simulink model "LPV_control"  (R2023a)
settings: Solver=VariableStepAuto  StartTime=0.0  StopTime=30  RelTol=1e-3
values from neighbouring files (symbols this model uses):
  Ad = [-1/t_beta 0 ... (first row only)    [calc_KMax.m]    (also in calc_Kmin.m; modelo.m)
  C = [1 0 ... (first row only)    [modelo.m]
  D = [0 0;0 0]    [modelo.m]
  Ed = [k_beta/t_beta ... (first row only)    [calc_KMax.m]    (also in calc_Kmin.m; modelo.m)
  x0 = [0, 0]    [modelo.m]
undefined symbols (not defined in the file or in its folder): calc_A, calc_B, calc_E, calc_inv_B, sigbuilder_block
settings Model: Creator=Ferna  LastModifiedBy=Ferna

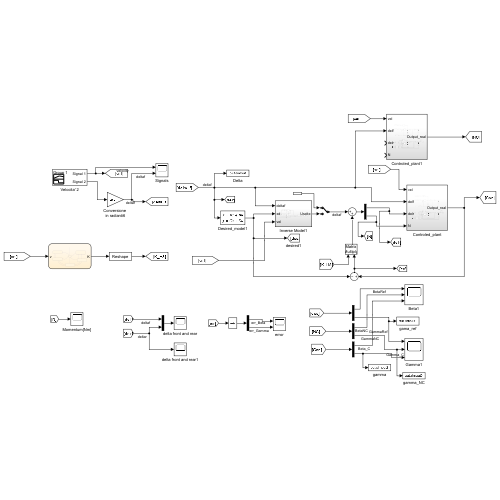
[thumbnail: Simulink's stored preview of the top-level diagram]
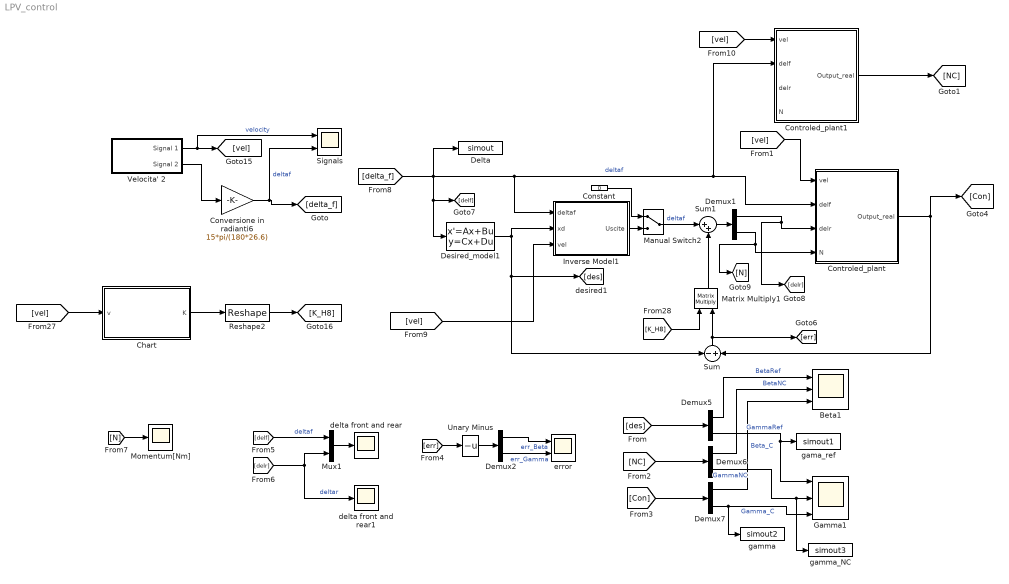
== system LPV_control ==
  Beta1 : Scope  NumInputPorts=3
  Chart : Stateflow chart  TreatAsAtomicUnit=on
  Constant : Constant  Value=0
  Controled_plant : Subsystem
  Controled_plant1 : Subsystem
  Conversione in radianti6 : Gain  Gain=15*pi/(180*26.6)
  Delta : ToWorkspace  VariableName=simout  SaveFormat=Timeseries  SampleTime=-1
  Demux{1..2,5..7} (5 alike) : Demux  Outputs=2
  Desired_model1 : StateSpace  A=Ad  B=Ed  C=[1,0;0,1]  D=zeros(2,1)  InitialCondition=0
  Gamma1 : Scope  NumInputPorts=3
  Inverse Model1 : Subsystem
  Manual Switch2 : ManualSwitch
  Matrix Multiply1 : Product  Multiplication=Matrix(*)
  Momentum[Nm] : Scope
  Mux1 : Mux  Inputs=2
  Reshape2 : Reshape  OutputDimensionality=Customize  OutputDimensions=[2,2]
  Signals : Scope  NumInputPorts=2
  Sum : Sum  Inputs=-|+
  Sum1 : Sum  Inputs=|++
  Unary Minus : UnaryMinus
  Velocita' 2 : Subsystem  Tag=STV Subsys  LoadFcn=sigbuilder_block('load');  StartFcn=sigbuilder_block('start');  StopFcn=sigbuilder_block('stop');  ClipboardFcn=sigbuilder_block('clipboard');  mask(Sigbuilder block){tuvar=[0:10]}
      mask help: Simulink:masks:SigbuilderBlock_MD
      mask init:
      | if ~strcmp(get_param(bdroot(gcbh),'SimulationStatus'),'stopped') tuvar = sigbuilder_block('maskInit'); end
      settings: CopyFcn=sigbuilder_block('copy');  DeleteFcn=sigbuilder_block('delete');  ModelCloseFcn=sigbuilder_block('modelClose');  PreSaveFcn=sigbuilder_block('preSave');  PauseFcn=sigbuilder_block('pause');  ContinueFcn=sigbuilder_block('continue');  NameChangeFcn=sigbuilder_block('namechange');  OpenFcn=sigbuilder_block('open',[5.4 36 1141.2 516.6 ]);  CloseFcn=sigbuilder_block('close');
      mask Display: plot(0, 0, 100, 100,[2, 2, 32, 32, 2], [68, 8, 8, 68, 68],[32, 2], [38, 38], [32, 19, 2],[53, 60, 44], [32, 17, 17, 2],[16, 16, 31, 31]);txt = getActiveGroup(gcbh);text(2, 100, txt,'verticalAlignment', 'top');
  delta front and rear : Scope
  delta front and rear1 : Scope
  error : Scope  NumInputPorts=2
  gama_ref : ToWorkspace  VariableName=simout1  SaveFormat=Timeseries  SampleTime=-1
  gamma : ToWorkspace  VariableName=simout2  SaveFormat=Timeseries  SampleTime=-1
  gamma_NC : ToWorkspace  VariableName=simout3  SaveFormat=Timeseries  SampleTime=-1
  wires:
  Conversione in radianti6/1 -> Signals/2, [delta_f]  "deltaf"
  Velocita' 2/2(Signal 2) -> Conversione in radianti6/1
  Demux5/2 -> gama_ref/1, Gamma1/1  "GammaRef"
  [N] -> Momentum[Nm]/1
  [delf] -> Mux1/1  "deltaf"
  Demux2/2 -> error/2  "err_Gamma"
  [delta_f] -> [delf], Desired_model1/1, Delta/1, Inverse Model1/1(deltaf), Controled_plant1/2(delf), Controled_plant/2(delf)  "deltaf"
  Demux2/1 -> error/1  "err_Beta"
  Mux1/1 -> delta front and rear/1
  Unary Minus/1 -> Demux2/1
  Sum1/1 -> Demux1/1
  Demux5/1 -> Beta1/1  "BetaRef"
  Demux6/1 -> Beta1/2  "BetaNC"
  [Con] -> Demux7/1
  [err] -> Unary Minus/1
  Demux1/1 -> [delr], Controled_plant/3(delr)
  [NC] -> Demux6/1
  Desired_model1/1 -> Inverse Model1/2(xd), Sum/1, [des]
  Demux1/2 -> [N], Controled_plant/4(N)
  Demux7/2 -> gamma/1, Gamma1/3  "Gamma_C"
  [delr] -> Mux1/2, delta front and rear1/1  "deltar"
  Demux7/1 -> Beta1/3  "Beta_C"
  [des] -> Demux5/1
  Controled_plant/1(Output_real) -> [Con], Sum/2
  Demux6/2 -> gamma_NC/1, Gamma1/2  "GammaNC"
  [vel] -> Controled_plant/1(vel)
  Velocita' 2/1(Signal 1) -> Signals/1, [vel]  "velocity"
  [vel] -> Inverse Model1/3(vel)
  Inverse Model1/1(Uscite) -> Manual Switch2/2
  Constant/1 -> Manual Switch2/1
  Manual Switch2/1 -> Sum1/1  "deltaf"
  Reshape2/1 -> [K_H8]
  [vel] -> Chart/1(v)
  Chart/1(K) -> Reshape2/1
  [K_H8] -> Matrix Multiply1/1
  Sum/1 -> Matrix Multiply1/2, [err]
  Matrix Multiply1/1 -> Sum1/2
  Controled_plant1/1(Output_real) -> [NC]
  [vel] -> Controled_plant1/1(vel)

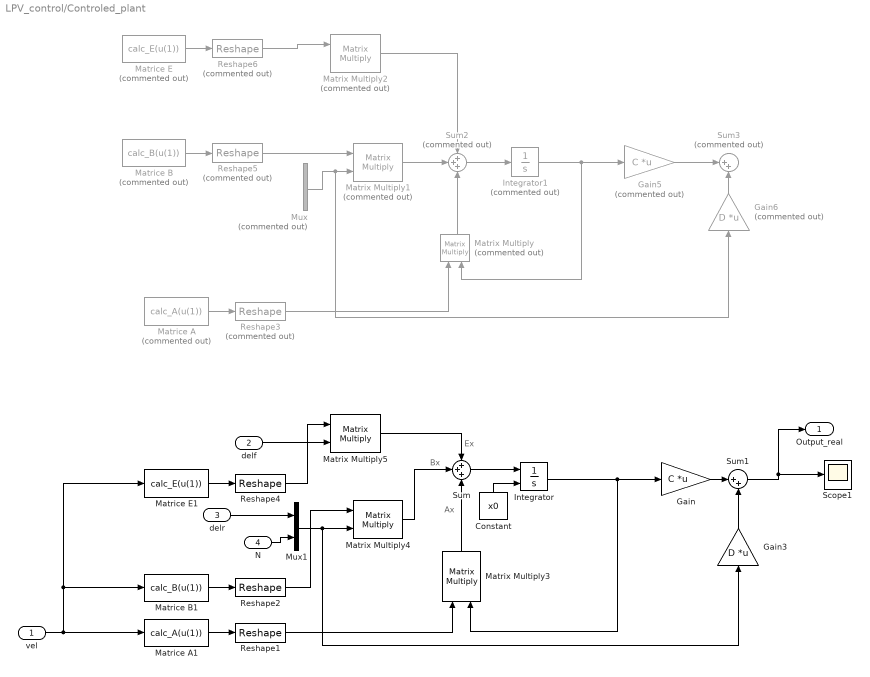
== system LPV_control/Controled_plant ==
  note: Ex
  note: Bx
  note: Ax
  vel : Inport
  delf : Inport  Port=2
  delr : Inport  Port=3
  N : Inport  Port=4
  Constant : Constant  Value=x0
  Gain : Gain  Gain=C  Multiplication=Matrix(K*u)
  Gain3 : Gain  Gain=D  Multiplication=Matrix(K*u)
  Gain5 : Gain  Commented=on  Gain=C  Multiplication=Matrix(K*u)
  Gain6 : Gain  Commented=on  Gain=D  Multiplication=Matrix(K*u)
  Integrator : Integrator  InitialConditionSource=external
  Integrator1 : Integrator  Commented=on  InitialCondition=x0
  Matrice A : MATLABFcn  Commented=on  MATLABFcn=calc_A(u(1))
  Matrice A1 : MATLABFcn  MATLABFcn=calc_A(u(1))
  Matrice B : MATLABFcn  Commented=on  MATLABFcn=calc_B(u(1))
  Matrice B1 : MATLABFcn  MATLABFcn=calc_B(u(1))
  Matrice E : MATLABFcn  Commented=on  MATLABFcn=calc_E(u(1))
  Matrice E1 : MATLABFcn  MATLABFcn=calc_E(u(1))
  Matrix Multiply : Product  Commented=on  Multiplication=Matrix(*)
  Matrix Multiply1 : Product  Commented=on  Multiplication=Matrix(*)
  Matrix Multiply2 : Product  Commented=on  Multiplication=Matrix(*)
  Matrix Multiply3 : Product  Multiplication=Matrix(*)
  Matrix Multiply4 : Product  Multiplication=Matrix(*)
  Matrix Multiply5 : Product  Multiplication=Matrix(*)
  Mux : Mux  Commented=on  Inputs=2
  Mux1 : Mux  Inputs=2
  Reshape1 : Reshape  OutputDimensionality=Customize  OutputDimensions=[2,2]
  Reshape2 : Reshape  OutputDimensionality=Customize  OutputDimensions=[2,2]
  Reshape3 : Reshape  Commented=on  OutputDimensionality=Customize  OutputDimensions=[2,2]
  Reshape4 : Reshape  OutputDimensionality=Customize  OutputDimensions=[2,1]
  Reshape5 : Reshape  Commented=on  OutputDimensionality=Customize  OutputDimensions=[2,2]
  Reshape6 : Reshape  Commented=on  OutputDimensionality=Customize  OutputDimensions=[2,1]
  Scope1 : Scope
  Sum : Sum  Inputs=+++
  Sum1 : Sum  Inputs=|++
  Sum2 : Sum  Commented=on  Inputs=+++
  Sum3 : Sum  Commented=on  Inputs=|++
  Output_real : Outport
  wires:
  Matrice E/1 -> Reshape6/1
  Reshape6/1 -> Matrix Multiply2/1
  Matrix Multiply1/1 -> Sum2/2
  Mux/1 -> Gain6/1, Matrix Multiply1/2
  Reshape3/1 -> Matrix Multiply/1
  Matrice A/1 -> Reshape3/1
  Gain5/1 -> Sum3/1
  Gain6/1 -> Sum3/2
  Integrator1/1 -> Gain5/1, Matrix Multiply/2
  Sum2/1 -> Integrator1/1
  Matrix Multiply2/1 -> Sum2/1
  Matrix Multiply/1 -> Sum2/3
  Matrice B/1 -> Reshape5/1
  Reshape5/1 -> Matrix Multiply1/1
  Matrix Multiply3/1 -> Sum/3
  delf/1 -> Matrix Multiply5/2
  Mux1/1 -> Gain3/1, Matrix Multiply4/2
  Gain3/1 -> Sum1/2
  Reshape2/1 -> Matrix Multiply4/1
  Matrix Multiply5/1 -> Sum/1
  Matrice A1/1 -> Reshape1/1
  Matrice E1/1 -> Reshape4/1
  Gain/1 -> Sum1/1
  vel/1 -> Matrice A1/1, Matrice E1/1, Matrice B1/1
  Sum/1 -> Integrator/1
  Reshape4/1 -> Matrix Multiply5/1
  Matrix Multiply4/1 -> Sum/2
  Integrator/1 -> Matrix Multiply3/2, Gain/1
  delr/1 -> Mux1/1
  Reshape1/1 -> Matrix Multiply3/1
  Matrice B1/1 -> Reshape2/1
  Constant/1 -> Integrator/2
  Sum1/1 -> Output_real/1, Scope1/1
  N/1 -> Mux1/2

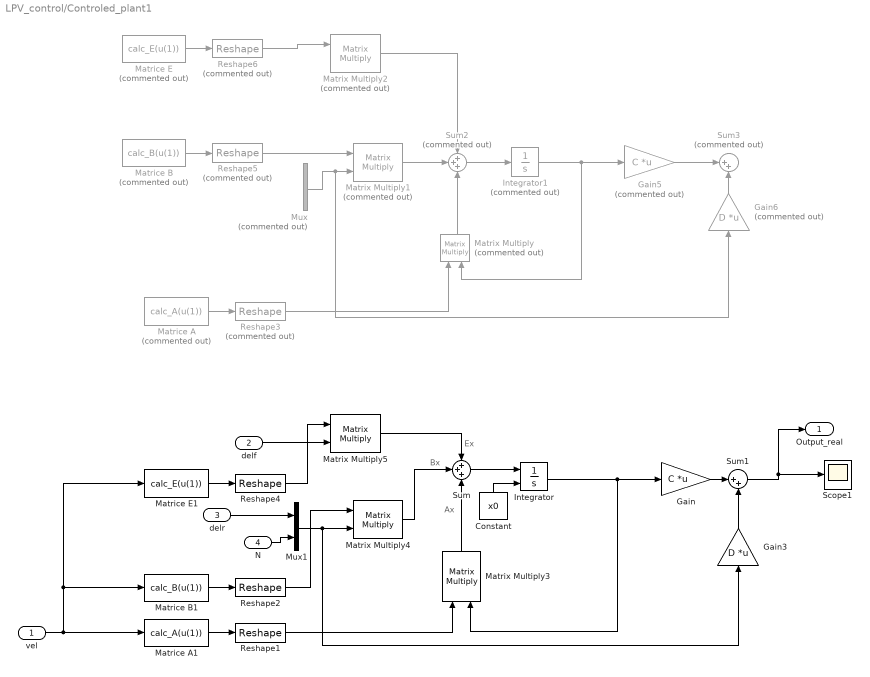
== system LPV_control/Controled_plant1 ==
  note: Ax
  note: Bx
  note: Ex
  vel : Inport
  delf : Inport  Port=2
  delr : Inport  Port=3
  N : Inport  Port=4
  Constant : Constant  Value=x0
  Gain : Gain  Gain=C  Multiplication=Matrix(K*u)
  Gain3 : Gain  Gain=D  Multiplication=Matrix(K*u)
  Gain5 : Gain  Commented=on  Gain=C  Multiplication=Matrix(K*u)
  Gain6 : Gain  Commented=on  Gain=D  Multiplication=Matrix(K*u)
  Integrator : Integrator  InitialConditionSource=external
  Integrator1 : Integrator  Commented=on  InitialCondition=x0
  Matrice A : MATLABFcn  Commented=on  MATLABFcn=calc_A(u(1))
  Matrice A1 : MATLABFcn  MATLABFcn=calc_A(u(1))
  Matrice B : MATLABFcn  Commented=on  MATLABFcn=calc_B(u(1))
  Matrice B1 : MATLABFcn  MATLABFcn=calc_B(u(1))
  Matrice E : MATLABFcn  Commented=on  MATLABFcn=calc_E(u(1))
  Matrice E1 : MATLABFcn  MATLABFcn=calc_E(u(1))
  Matrix Multiply : Product  Commented=on  Multiplication=Matrix(*)
  Matrix Multiply1 : Product  Commented=on  Multiplication=Matrix(*)
  Matrix Multiply2 : Product  Commented=on  Multiplication=Matrix(*)
  Matrix Multiply3 : Product  Multiplication=Matrix(*)
  Matrix Multiply4 : Product  Multiplication=Matrix(*)
  Matrix Multiply5 : Product  Multiplication=Matrix(*)
  Mux : Mux  Commented=on  Inputs=2
  Mux1 : Mux  Inputs=2
  Reshape1 : Reshape  OutputDimensionality=Customize  OutputDimensions=[2,2]
  Reshape2 : Reshape  OutputDimensionality=Customize  OutputDimensions=[2,2]
  Reshape3 : Reshape  Commented=on  OutputDimensionality=Customize  OutputDimensions=[2,2]
  Reshape4 : Reshape  OutputDimensionality=Customize  OutputDimensions=[2,1]
  Reshape5 : Reshape  Commented=on  OutputDimensionality=Customize  OutputDimensions=[2,2]
  Reshape6 : Reshape  Commented=on  OutputDimensionality=Customize  OutputDimensions=[2,1]
  Scope1 : Scope
  Sum : Sum  Inputs=+++
  Sum1 : Sum  Inputs=|++
  Sum2 : Sum  Commented=on  Inputs=+++
  Sum3 : Sum  Commented=on  Inputs=|++
  Output_real : Outport
  wires:
  N/1 -> Mux1/2
  Sum1/1 -> Scope1/1, Output_real/1
  Constant/1 -> Integrator/2
  Matrice B1/1 -> Reshape2/1
  Reshape1/1 -> Matrix Multiply3/1
  delr/1 -> Mux1/1
  Integrator/1 -> Gain/1, Matrix Multiply3/2
  Matrix Multiply4/1 -> Sum/2
  Reshape4/1 -> Matrix Multiply5/1
  Sum/1 -> Integrator/1
  vel/1 -> Matrice B1/1, Matrice E1/1, Matrice A1/1
  Gain/1 -> Sum1/1
  Matrice E1/1 -> Reshape4/1
  Matrice A1/1 -> Reshape1/1
  Matrix Multiply5/1 -> Sum/1
  Reshape2/1 -> Matrix Multiply4/1
  Gain3/1 -> Sum1/2
  Mux1/1 -> Matrix Multiply4/2, Gain3/1
  delf/1 -> Matrix Multiply5/2
  Matrix Multiply3/1 -> Sum/3
  Reshape5/1 -> Matrix Multiply1/1
  Matrice B/1 -> Reshape5/1
  Matrix Multiply/1 -> Sum2/3
  Matrix Multiply2/1 -> Sum2/1
  Sum2/1 -> Integrator1/1
  Integrator1/1 -> Matrix Multiply/2, Gain5/1
  Gain6/1 -> Sum3/2
  Gain5/1 -> Sum3/1
  Matrice A/1 -> Reshape3/1
  Reshape3/1 -> Matrix Multiply/1
  Mux/1 -> Matrix Multiply1/2, Gain6/1
  Matrix Multiply1/1 -> Sum2/2
  Reshape6/1 -> Matrix Multiply2/1
  Matrice E/1 -> Reshape6/1

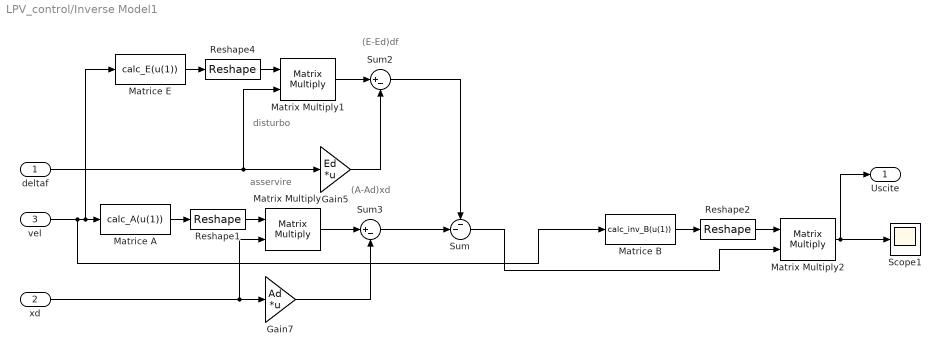
== system LPV_control/Inverse Model1 ==
  note: disturbo
  note: asservire
  note: (E-Ed)df
  note: (A-Ad)xd
  deltaf : Inport
  xd : Inport  Port=2  PortDimensions=2
  vel : Inport  Port=3  PortDimensions=1
  Gain5 : Gain  Gain=Ed  Multiplication=Matrix(K*u)
  Gain7 : Gain  Gain=Ad  Multiplication=Matrix(K*u)
  Matrice A : MATLABFcn  MATLABFcn=calc_A(u(1))
  Matrice B : MATLABFcn  MATLABFcn=calc_inv_B(u(1))
  Matrice E : MATLABFcn  MATLABFcn=calc_E(u(1))
  Matrix Multiply : Product  Multiplication=Matrix(*)
  Matrix Multiply1 : Product  Multiplication=Matrix(*)
  Matrix Multiply2 : Product  Multiplication=Matrix(*)
  Reshape1 : Reshape  OutputDimensionality=Customize  OutputDimensions=[2,2]
  Reshape2 : Reshape  OutputDimensionality=Customize  OutputDimensions=[2,2]
  Reshape4 : Reshape  OutputDimensionality=Customize  OutputDimensions=[2,1]
  Scope1 : Scope
  Sum : Sum  Inputs=--|
  Sum2 : Sum  Inputs=|+-
  Sum3 : Sum  Inputs=|+-
  Uscite : Outport
  wires:
  xd/1 -> Gain7/1, Matrix Multiply/2
  deltaf/1 -> Matrix Multiply1/2, Gain5/1
  Matrix Multiply1/1 -> Sum2/1
  Gain5/1 -> Sum2/2
  Gain7/1 -> Sum3/2
  Matrix Multiply/1 -> Sum3/1
  Matrice A/1 -> Reshape1/1
  Reshape1/1 -> Matrix Multiply/1
  vel/1 -> Matrice B/1, Matrice E/1, Matrice A/1
  Matrice E/1 -> Reshape4/1
  Reshape4/1 -> Matrix Multiply1/1
  Sum2/1 -> Sum/1
  Sum3/1 -> Sum/2
  Matrice B/1 -> Reshape2/1
  Reshape2/1 -> Matrix Multiply2/1
  Sum/1 -> Matrix Multiply2/2
  Matrix Multiply2/1 -> Uscite/1, Scope1/1

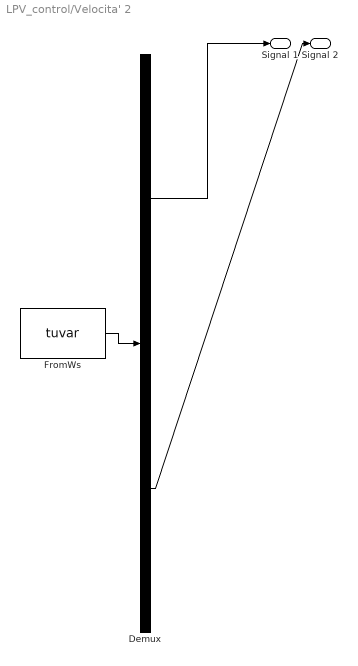
== system LPV_control/Velocita' 2 ==
  Demux : Demux  Tag=STV Demux  Outputs=2
      settings: DisplayOption=none
  FromWs : FromWorkspace  Tag=STV FromWs  VariableName=tuvar
      SigBuilderData=|
      | common.afterFinalStr = 'Extrapolate'
      | common.sampleTime = 0
      | dataSet.timeRange = [0 34]
      | dataSet.name = 'Group 1'
      | sbobj.Groups.Name = 'Group 1'
      | sbobj.Groups.Signals(1).Name = 'Signal 1'
      | sbobj.Groups.Signals(1).XData = [0 1 4 6 10 12 16 18 22 24 34]
      | sbobj.Groups.Signals(1).YData = [51 51 51 62 62 72 72 85 85 95 95]
      | sbobj.Groups.Signals(2).Name = 'Signal 2'
      | sbobj.Groups.Signals(2).XData = [0 1 1.25 1.5 1.75 2 2.25 2.5 2.75 3 4 6 7 7.25 7.5 7.75 8 8.25 8.5 8.75 9 10 12 13 13.25 13.5 13.75 14 14.25 14.5 14.75 15 16 19 19.25 19.5 19.75 20 20.25 20.5 20.75 21 25 25.25 25.5 25.75 26 26.25 26.5 26.75 27 34]
      | sbobj.Groups.Signals(2).YData = [0 0 0.7 1 0.7 0 -0.7 -1 -0.7 0 0 0 0 0.7 1 0.7 0 -0.7 -1 -0.7 0 0 0 0 0.7 1 0.7 0 -0.7 -1 -0.7 0 0 0 0.7 1 0.7 0 -0.7 -1 -0.7 0 0 0.7 1 0.7 0 -0.7 -1 -0.7 0 0]
      | sbobj.Groups.TimeRange = [0 34]
  Signal 1 : Outport  Tag=STV Outport
  Signal 2 : Outport  Tag=STV Outport  Port=2
  wires:
  FromWs/1 -> Demux/1
  Demux/1 -> Signal 1/1
  Demux/2 -> Signal 2/1

== stateflow chart LPV_control/Chart ==
  note: Stato di neutro
  state S1
    entry: rho=(v-50)/(60-50);
    entry:Kmi_1=ml('calc_Kmin(%d%)',50);
    entry:KMa_1=ml('calc_KMax(%d%)',60);
    entry:K=(1-rho)*Kmi_1+rho*KMa_1;
    c1=v;
  state S5
    entry: rho=(v-90)/(100-90);
    entry:Kmi_5=ml('calc_Kmin(%d%)',90);
    entry:KMa_5=ml('calc_KMax(%d%)',100);
    entry:K=(1-rho)*Kmi_5+rho*KMa_5;
    c1=v;
  state S0
  state S2
    entry: rho=(v-60)/(70-60);
    entry:Kmi_2=ml('calc_Kmin(%d%)',60);
    entry:KMa_2=ml('calc_KMax(%d%)',70);
    entry:K=(1-rho)*Kmi_2+rho*KMa_2;
    c1=v;
  state S4
    entry: rho=(v-80)/(90-80);
    entry:Kmi_4=ml('calc_Kmin(%d%)',80);
    entry:KMa_4=ml('calc_KMax(%d%)',90);
    entry:K=(1-rho)*Kmi_4+rho*KMa_4;
    c1=v;
  state S3
    entry: rho=(v-70)/(80-70);
    entry:Kmi_3=ml('calc_Kmin(%d%)',70);
    entry:KMa_3=ml('calc_KMax(%d%)',80);
    entry:K=(1-rho)*Kmi_3+rho*KMa_3;
    c1=v;
  (default) -> S0
  S0 -> S1 [order 1] : [v>50 && v<=60]
  S0 -> S5 [order 2] : [v>90 && v<=100]
  S1 -> S2 : [v>60]
  S2 -> S1 [order 1] : [v<=60]
  S5 -> S4 : [v<=90]
  S4 -> S5 [order 1] : [v>90]
  S0 -> S2 [order 5] : [v>60 && v<=70]
  S0 -> S3 [order 4] : [v>70 && v<=80]
  S0 -> S4 [order 3] : [v>80 && v<=90]
  S2 -> S3 [order 2] : [v>70]
  S3 -> S2 [order 2] : [v<=70]
  S4 -> S3 [order 2] : [v<=80]
  S3 -> S4 [order 1] : [v>80]
  data: v input double; c1 local double; c2 local double; K output double size=4; Kmi_1 local double size=4; KMa_1 local double size=4; Kmi_2 local double size=4; KMa_2 local double size=4; Kmi_3 local double size=4; KMa_3 local double size=4; KMa_4 local double size=4; KMa_5 local double size=4; KMa_6 local double size=4; KMa_7 local double size=4; Kmi_4 local double size=4; Kmi_5 local double size=4; Kmi_6 local double size=4; Kmi_7 local double size=4; rho local double
